simulink model "simulink_1"  (R2013a)
settings: Solver=ode45  StartTime=0.0  StopTime=10.0  RelTol=1e-3
settings Model: Creator=alper pc  LastModifiedBy=alper pc

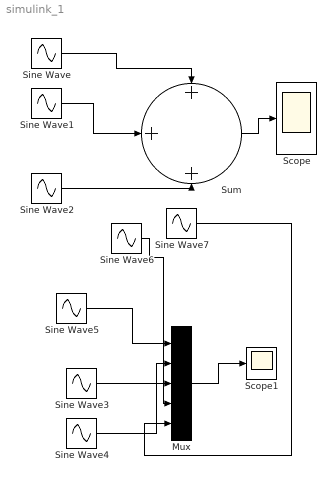
== system simulink_1 ==
  Mux : Mux  Inputs=5
  Scope : Scope
  Scope1 : Scope
  Sine Wave : Sin  SampleTime=0
  Sine Wave1 : Sin  Amplitude=6  SampleTime=0
  Sine Wave2 : Sin  Amplitude=7  SampleTime=0
  Sine Wave3 : Sin  Amplitude=5  SampleTime=0
  Sine Wave4 : Sin  Amplitude=3  SampleTime=0
  Sine Wave5 : Sin  SampleTime=0
  Sine Wave6 : Sin  Amplitude=8  SampleTime=0
  Sine Wave7 : Sin  Amplitude=9  SampleTime=0
  Sum : Sum  Inputs=+++
  wires:
  Sine Wave/1 -> Sum/1
  Sine Wave1/1 -> Sum/2
  Sine Wave2/1 -> Sum/3
  Sum/1 -> Scope/1
  Sine Wave5/1 -> Mux/1
  Sine Wave3/1 -> Mux/2
  Sine Wave4/1 -> Mux/3
  Mux/1 -> Scope1/1
  Sine Wave6/1 -> Mux/4
  Sine Wave7/1 -> Mux/5
